simulink model "untitled"  (R2023b)
settings: Solver=VariableStepAuto  StartTime=0.0  StopTime=10.0  RelTol=1e-3
libraries: simulink x2
settings Model: Creator=ander  LastModifiedBy=ander

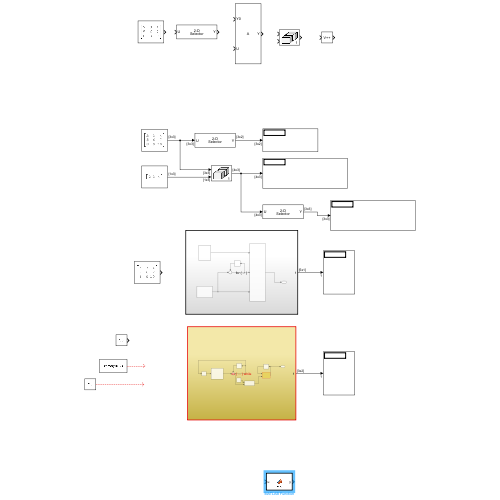
[thumbnail: Simulink's stored preview of the top-level diagram]
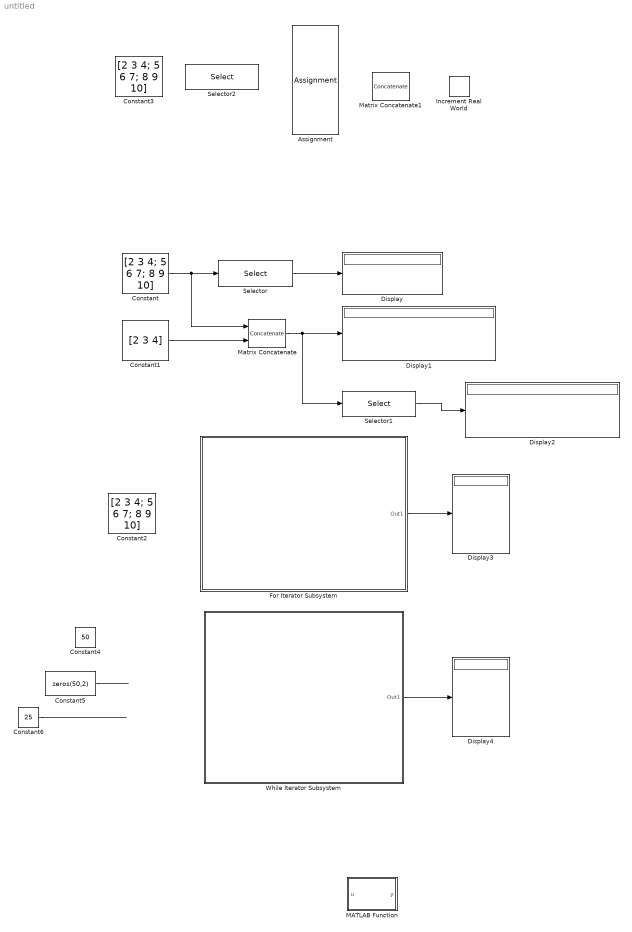
== system untitled ==
  Assignment : Assignment  DiagnosticForDimensions=Warning  IndexOptions=Index vector (dialog)  Indices=1  OutputSizes=1
  Constant : Constant  Value=[2 3 4; 5 6 7; 8 9 10]
  Constant1 : Constant  Value=[2 3 4]  VectorParams1D=off
  Constant2 : Constant  Value=[2 3 4; 5 6 7; 8 9 10]
  Constant3 : Constant  Value=[2 3 4; 5 6 7; 8 9 10]
  Constant4 : Constant  Value=50
  Constant5 : Constant  Value=zeros(50,2)
  Constant6 : Constant  Value=25
  Display{,1..4} (5 alike) : Display
  For Iterator Subsystem : Subsystem  TreatAsAtomicUnit=on
  Increment Real World : simulink/Additional Math & Discrete/Additional Math: Increment - Decrement/Increment Real World
  MATLAB Function : MATLAB Function  TreatAsAtomicUnit=on
  Matrix Concatenate : Concatenate  Mode=Multidimensional array
  Matrix Concatenate1 : Concatenate  Mode=Multidimensional array
  Selector : Selector  NumberOfDimensions=2  InputPortWidth=3  IndexOptions=Index vector (dialog),Index vector (dialog)  Indices=[1 2 3],[1 3]  OutputSizes=1,1
  Selector1 : Selector  NumberOfDimensions=2  InputPortWidth=3  IndexOptions=Index vector (dialog),Select all  Indices=[1 2 3],[1 3]  OutputSizes=1,1
  Selector2 : Selector  NumberOfDimensions=2  InputPortWidth=3  IndexOptions=Index vector (dialog),Index vector (dialog)  Indices=[1 2 3],[1 3]  OutputSizes=1,1
  While Iterator Subsystem : Subsystem  TreatAsAtomicUnit=on
  wires:
  Constant/1 -> Matrix Concatenate/1, Selector/1
  Selector/1 -> Display/1
  Constant1/1 -> Matrix Concatenate/2
  Matrix Concatenate/1 -> Selector1/1, Display1/1
  Selector1/1 -> Display2/1
  For Iterator Subsystem/1(Out1) -> Display3/1
  While Iterator Subsystem/1(Out1) -> Display4/1
  Constant6/1 -> ?
  Constant5/1 -> ?

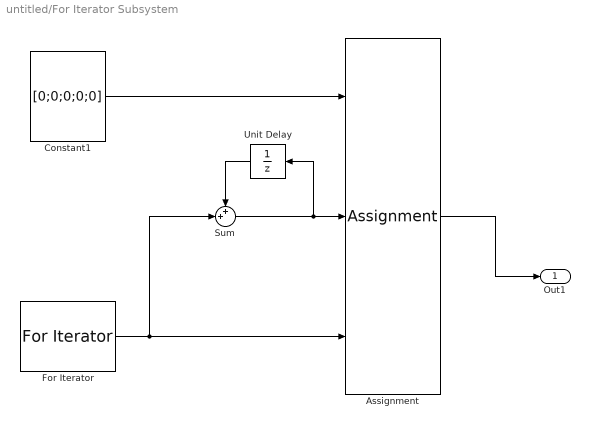
== system untitled/For Iterator Subsystem ==
  Assignment : Assignment  NumberOfDimensions=2  DiagnosticForDimensions=Warning  IndexOptions=Index vector (port),Index vector (dialog)  Indices=1,1  OutputSizes=1,1
  Constant1 : Constant  Value=[0;0;0;0;0]  VectorParams1D=off
  For Iterator : ForIterator  ResetStates=reset  IterationVariableDataType=double
  Sum : Sum  Inputs=++|
  Unit Delay : UnitDelay  SampleTime=-1  HasFrameUpgradeWarning=on
  Out1 : Outport
  wires:
  Constant1/1 -> Assignment/1
  Assignment/1 -> Out1/1
  For Iterator/1 -> Sum/2, Assignment/3
  Sum/1 -> Unit Delay/1, Assignment/2
  Unit Delay/1 -> Sum/1

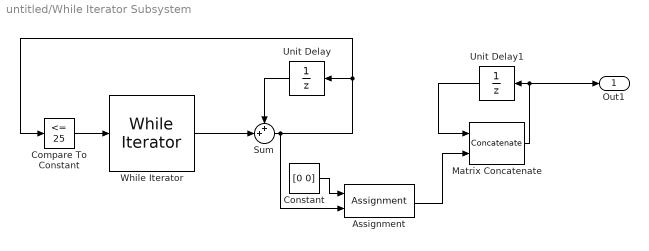
== system untitled/While Iterator Subsystem ==
  Assignment : Assignment  NumberOfDimensions=2  DiagnosticForDimensions=Warning  IndexOptions=Index vector (dialog),Index vector (dialog)  Indices=1,1  OutputSizes=1,1
  Compare To Constant : simulink/Logic and Bit Operations/Compare To Constant  relop=<=  const=25  OutDataTypeStr=boolean
  Constant : Constant  Value=[0 0]  VectorParams1D=off
  Matrix Concatenate : Concatenate  Mode=Multidimensional array
  Sum : Sum  Inputs=++|
  Unit Delay : UnitDelay  SampleTime=-1  HasFrameUpgradeWarning=on
  Unit Delay1 : UnitDelay  InitialCondition=zeros(2,2)  SampleTime=-1  HasFrameUpgradeWarning=on
  While Iterator : WhileIterator  MaxIters=-1  WhileBlockType=do-while  ResetStates=reset  ShowIterationPort=on  OutputDataType=double
  Out1 : Outport
  wires:
  Compare To Constant/1 -> While Iterator/1
  Unit Delay/1 -> Sum/1
  While Iterator/1 -> Sum/2
  Unit Delay1/1 -> Matrix Concatenate/1
  Matrix Concatenate/1 -> Out1/1, Unit Delay1/1
  Sum/1 -> Assignment/2, Compare To Constant/1, Unit Delay/1
  Constant/1 -> Assignment/1
  Assignment/1 -> Matrix Concatenate/2

== matlab function untitled/MATLAB Function ==
  data: u input; y output
function y = fcn(u)

y = u;
